simulink model "inv_opt"  (R2019a)
settings: Solver=VariableStepAuto  StartTime=0.0  StopTime=10.0  RelTol=1e-3
settings Model: Creator=shobhitvoleti  LastModifiedBy=shobhitvoleti

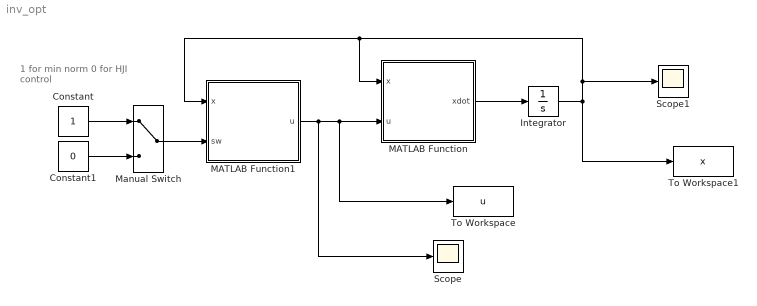
== system inv_opt ==
  note: 1 for min norm
      | 0 for HJI control
  Constant : Constant
  Constant1 : Constant  Value=0
  Integrator : Integrator  InitialCondition=2
  MATLAB Function : MATLAB Function  TreatAsAtomicUnit=on
  MATLAB Function1 : MATLAB Function  TreatAsAtomicUnit=on
  Manual Switch : ManualSwitch
  Scope : Scope
  Scope1 : Scope
  To Workspace : ToWorkspace  VariableName=u  SampleTime=-1
  To Workspace1 : ToWorkspace  VariableName=x  SampleTime=-1
  wires:
  MATLAB Function/1(xdot) -> Integrator/1
  Integrator/1 -> Scope1/1, MATLAB Function1/1(x), MATLAB Function/1(x), To Workspace1/1
  MATLAB Function1/1(u) -> Scope/1, To Workspace/1, MATLAB Function/2(u)
  Manual Switch/1 -> MATLAB Function1/2(sw)
  Constant/1 -> Manual Switch/1
  Constant1/1 -> Manual Switch/2

== matlab function inv_opt/MATLAB Function1 ==
  data: x input; u output; sw input
function u = fcn(x,sw)


if sw == 1
   
    if x^2 < 2
      u = x^3 - 2*x;
    else
      u = 0;
    end

else
    u = x^3 -x -x*sqrt(x^4 - 2*x^2 + 2);

end

== matlab function inv_opt/MATLAB Function ==
  settings: updateMethod=DISCRETE
  data: x input; u input; xdot output
function xdot = fcn(x,u)

%w = randi([-1 1],1,1);

w = 1;
xdot = -x^3 + u +w*x;
